simulink library "gs_prediction_lib"  (R2016b)
settings: Solver=ode45  StartTime=0.0  StopTime=86400  RelTol=1e-3  EnableMultiTasking=on
undefined symbols (not defined in the file or in its folder): Earth, fsw_params, WGS84
libraries: aerolibtransform2 x1
settings Model: Creator=Taylor  LastModifiedBy=evich
settings DataIOCC: LimitDataPoints=on
settings OptimizationCC: LifeSpan=inf
settings DebuggingCC: AllowSymbolicDim=off  SFUnexpectedBacktrackingDiag=warning  SFNoUnconditionalDefaultTransitionDiag=warning  SFExecutionAtInitializationDiag=none
settings GRTTargetCC: TargetLangStandard=C89/C90 (ANSI)  GeneratePreprocessorConditionals=Disable all
settings ConfigComp: CovMetricSettings=dw  CovHtmlReporting=on  CovSaveCumulativeToWorkspaceVar=on  CovSaveSingleToWorkspaceVar=on  CovExternalEMLEnable=off

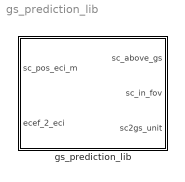
== system gs_prediction_lib ==
  gs_prediction_lib : Subsystem  TreatAsAtomicUnit=on
      settings: MinAlgLoopOccurrences=on  RTWFcnNameOpts=Use subsystem name  RTWFileNameOpts=Use subsystem name

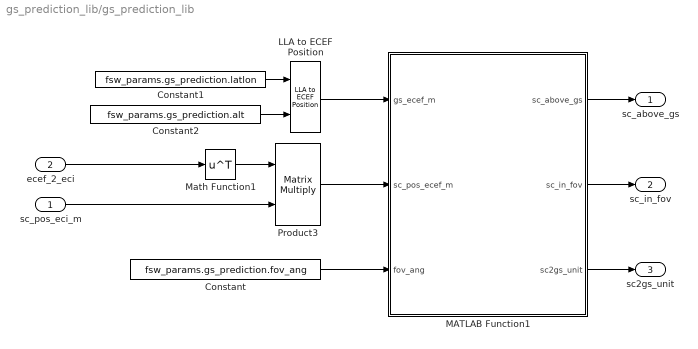
== system gs_prediction_lib/gs_prediction_lib ==
  sc_pos_eci_m : Inport
  ecef_2_eci : Inport  Port=2
  Constant : Constant  Value=fsw_params.gs_prediction.fov_ang  SampleTime=fsw_params.gs_prediction.sample_time_s
  Constant1 : Constant  Value=fsw_params.gs_prediction.latlon  SampleTime=fsw_params.gs_prediction.sample_time_s
  Constant2 : Constant  Value=fsw_params.gs_prediction.alt  SampleTime=fsw_params.gs_prediction.sample_time_s
  LLA to ECEF Position : aerolibtransform2/LLA to ECEF Position  units=Metric (MKS)  ptype=Earth (WGS84)  F=1/298.257223563  R=6378137
  MATLAB Function1 : MATLAB Function  TreatAsAtomicUnit=on
  Math Function1 : Math  Operator=transpose  SaturateOnIntegerOverflow=on
  Product3 : Product  Multiplication=Matrix(*)
  sc_above_gs : Outport
  sc_in_fov : Outport  Port=2
  sc2gs_unit : Outport  Port=3
  wires:
  sc_pos_eci_m/1 -> Product3/2
  Math Function1/1 -> Product3/1
  ecef_2_eci/1 -> Math Function1/1
  MATLAB Function1/1(sc_above_gs) -> sc_above_gs/1
  MATLAB Function1/3(sc2gs_unit) -> sc2gs_unit/1
  Product3/1 -> MATLAB Function1/2(sc_pos_ecef_m)
  MATLAB Function1/2(sc_in_fov) -> sc_in_fov/1
  Constant/1 -> MATLAB Function1/3(fov_ang)
  Constant1/1 -> LLA to ECEF Position/1
  Constant2/1 -> LLA to ECEF Position/2
  LLA to ECEF Position/1 -> MATLAB Function1/1(gs_ecef_m)

== matlab function gs_prediction_lib/MATLAB Function1 ==
  data: gs_ecef_m input; sc_above_gs output; sc_in_fov output; sc2gs_unit output; sc_pos_ecef_m input; fov_ang input
function [sc_above_gs,sc_in_fov,sc2gs_unit] = sc_above_gs(gs_ecef_m,sc_pos_ecef_m,fov_ang)
% Calculates if the ground station is in the field of view.

% Constants
TRUE        = 1;
FALSE       = 0;
% -----

% Main Function

% Remnant from sun_vector, may not be relevant here?
% gs_eci_km(3)  = gs_eci_km(3)/(sqrt(1 - ECCE2));
% sc_pos_eci_km(3)        = sc_pos_eci_km(3)/(sqrt(1 - ECCE2));

gs_vec     = gs_ecef_m;
sc_vec      = sc_pos_ecef_m;

%In ECI coordinates
sc2gs_unit  = (gs_vec - sc_vec)/norm(gs_vec - sc_vec);

% Determine if the sc is above the horizon in Seattle

sc2gs_gs_dot  = dot(sc2gs_unit,gs_vec)/norm(gs_vec);

% Check LoS
if sc2gs_gs_dot < 0
    ABOVE     = TRUE;
else
    ABOVE     = FALSE;
end

sc_above_gs = ABOVE;

pr = sc_vec - gs_vec;
fs = norm(pr)*cosd(fov_ang) - gs_vec'*pr/norm(gs_vec);
if (fs < 0)
    sc_in_fov = TRUE;
else
    sc_in_fov = FALSE;
end
